simulink subsystem "Normalize_Pose_Error"  (R2023a)
settings: Solver=VariableStepAuto  StartTime=0.0  StopTime=10.0  RelTol=1e-3
settings Model: Creator=hollis  LastModifiedBy=john

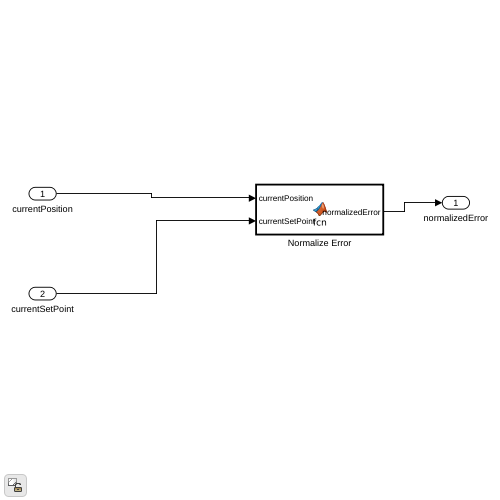
[thumbnail: Simulink's stored preview of the top-level diagram]
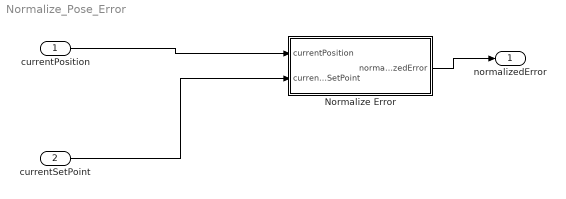
== system Normalize_Pose_Error ==
  currentPosition : Inport
  currentSetPoint : Inport  Port=2
  Normalize Error : MATLAB Function  TreatAsAtomicUnit=on
  normalizedError : Outport
  wires:
  currentPosition/1 -> Normalize Error/1(currentPosition)
  Normalize Error/1(normalizedError) -> normalizedError/1
  currentSetPoint/1 -> Normalize Error/2(currentSetPoint)

== matlab function Normalize_Pose_Error/Normalize Error ==
  data: currentPosition input; normalizedError output; currentSetPoint input
function normalizedError = fcn(currentPosition, currentSetPoint)

normalized = zeros(1,6);

normalized(1) = currentPosition(1) - currentSetPoint(1);
normalized(2) = currentPosition(2) - currentSetPoint(2);
normalized(3) = currentPosition(3) - currentSetPoint(3);

W2B = [currentPosition(7), currentPosition(4), currentPosition(5), currentPosition(6)];
setQuat = [currentSetPoint(7), -currentSetPoint(4), -currentSetPoint(5), -currentSetPoint(6)];


%Talos Heading in Body Frame
Tbody = [1,0,0,0];

%Transform from Body 2 World
B2W = [W2B(1), -W2B(2), -W2B(3), -W2B(4)] / (norm(W2B) ^ 2);

%Talos Heading in World Frame
TWorld = quatmultiply(Tbody, B2W);

%Talos Heading in World Frame Conjugate
TWorldI = [TWorld(1), -TWorld(2), -TWorld(3), -TWorld(4)];

%Current Yaw Error
eQuat = quatmultiply(setQuat, TWorldI);

% %axis Error
axisError = [eQuat(2), eQuat(3), eQuat(4)];
if(eQuat(1) < 0)
    axisError = -axisError;
end


normalized(4) = axisError(1);
normalized(5) = axisError(2);
normalized(6) = axisError(3);

normalizedError = normalized;
